simulink model "ex18_sfw_top"  (R2025a)
settings: Solver=FixedStepDiscrete  StartTime=0.0  StopTime=sfw_stop_s  FixedStep=sfw_sample_s  RelTol=1e-3
InitFcn:
  | model_dir = fileparts(get_param(bdroot, 'FileName'));if ~isempty(model_dir), addpath(model_dir); addpath(fullfile(model_dir, 'filterlib')); addpath(fullfile(model_dir, 'dialogs')); end;setup_ex18_sfw;
undefined symbols (not defined in the file or in its folder): gpr_rx_angle_deg, gpr_soil_fir, iq_lo_amp, iq_lo_hz, iq_lpf_num, physconst, rational, rf_z0_ohm, rx_down_if_bpf_den, rx_down_if_bpf_num, S, sfw_freq_hz, sfw_sample_s, sparameters, tap_lo_amp, tap_lo_hz, tap_up_bpf_den, tap_up_bpf_num
libraries: simrfV2elements x4, simrfV2util1 x4, simrfV2_lib x2
settings Model: Creator=31885  LastModifiedBy=31885
settings DataIOCC: SaveFormat=StructureWithTime  ReturnWorkspaceOutputs=off

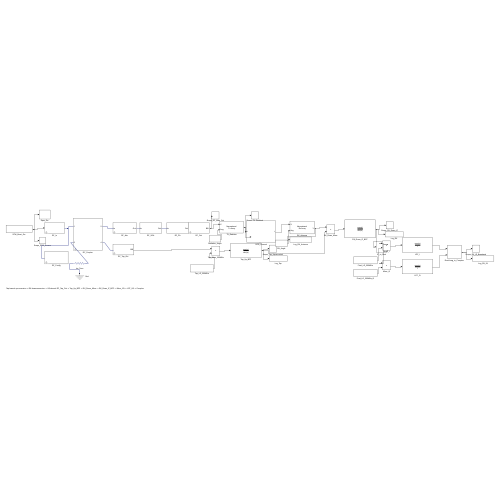
[thumbnail: Simulink's stored preview of the top-level diagram]
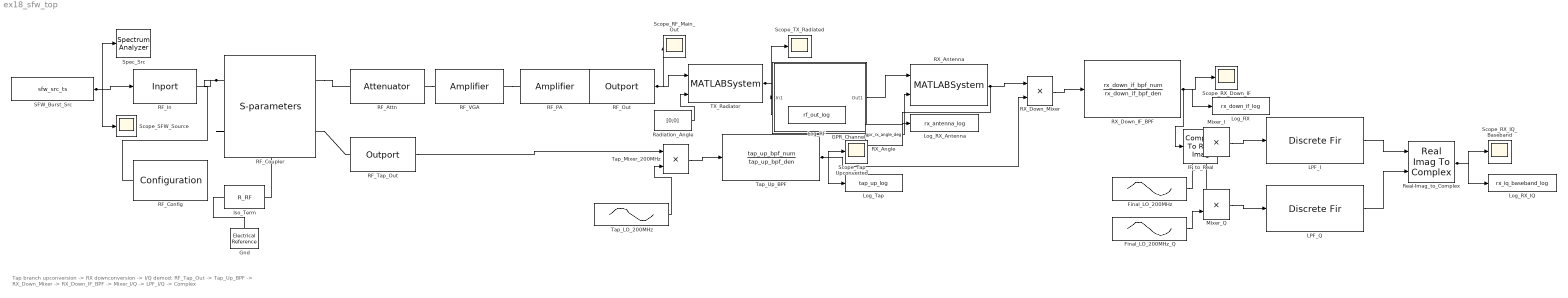
== system ex18_sfw_top ==
  note: Tap branch upconversion -> RX downconversion -> I/Q demod: RF_Tap_Out -> Tap_Up_BPF -> RX_Down_Mixer -> RX_Down_IF_BPF -> Mixer_I/Q -> LPF_I/Q -> Complex
  Final_LO_200MHz : Sin  Amplitude=iq_lo_amp  Frequency=2*pi*iq_lo_hz  SampleTime=sfw_sample_s
  Final_LO_200MHz_Q : Sin  Amplitude=iq_lo_amp  Frequency=2*pi*iq_lo_hz  Phase=-pi/2  SampleTime=sfw_sample_s
  GPR_Channel : Subsystem
  Gnd : simrfV2_lib/Elements/Electrical Reference
      settings: InternalSimscapePortConfiguration="{\"Bottom\":[],\"Left\":[{\"id\":\"V\",\"label\":\"\",\"type\":\"foundation.rf.circuitenvelope\"}],\"Right\":[],\"Top\":[]}"
  IF_to_Real : ComplexToRealImag
  Iso_Term : simrfV2_lib/Elements/R_RF  R=rf_z0_ohm Ohm
      settings: InternalSimscapePortConfiguration="{\"Bottom\":[],\"Left\":[{\"id\":\"p\",\"label\":\"+\",\"type\":\"foundation.rf.circuitenvelope\"}],\"Right\":[{\"id\":\"n\",\"label\":\"-\",\"type\":\"foundation.rf.circuitenvelope\"}],\"Top\":[]}"
  LPF_I : DiscreteFir  Coefficients=iq_lpf_num  SampleTime=sfw_sample_s
      settings: OpenFcn=ex18_filter_dialog(gcb);
  LPF_Q : DiscreteFir  Coefficients=iq_lpf_num  SampleTime=sfw_sample_s
      settings: OpenFcn=ex18_filter_dialog(gcb);
  Log_RF : ToWorkspace  VariableName=rf_out_log  SaveFormat=Structure With Time  SampleTime=-1
  Log_RX : ToWorkspace  VariableName=rx_down_if_log  SaveFormat=Structure With Time  SampleTime=-1
  Log_RX_Antenna : ToWorkspace  VariableName=rx_antenna_log  SaveFormat=Structure With Time  SampleTime=-1
  Log_RX_IQ : ToWorkspace  VariableName=rx_iq_baseband_log  SaveFormat=Structure With Time  SampleTime=-1
  Log_Tap : ToWorkspace  VariableName=tap_up_log  SaveFormat=Structure With Time  SampleTime=-1
  Mixer_I : Product  Inputs=**
  Mixer_Q : Product  Inputs=**
  RF_Attn : simrfV2elements/Attenuator  classname=attenuator  Att=rf_attn_db  Zin=rf_z0_ohm  Zout=rf_z0_ohm  AddNoise=on  InternalGrounding=on
  RF_Config : simrfV2util1/Configuration  AutoFreq=on  Tones=[] Hz  Harmonics=[]  NormalizeCarrierPower=on  SolverType=Auto  UseCCode=on  StepSize=sfw_sample_s s  AddNoise=on  defaultRNG=on  Seed=0  Temperature=290.0 K  SolverDelFlag=0  AbsTol=1e-6  RelTol=1e-3  MaxIter=10  ErrorEstimationType=2-norm over all variables  EnableInterpFilter=on  HiddenFIRfilterControllerParam=off  SmallSignalApprox=off  AllSimFreqs=on  SimFreqs=[] Hz  SimFreqsInternal=[]  SamplesPerFrame=1
  RF_Coupler : simrfV2elements/S-parameters  classname=sparam_element  DataSource=Network-parameters  File=unitygain.s2p  isNetworkObj=off  NetworkObject=sparameters('default.s2p')  Paramtype=S-parameters  Sparam=[0 0 0 0;0.70794578438413791 0 0 0;0 0 0 0;0.50118723362727224 0 0 0]  SparamFreq=145000000 Hz  SparamZ0=50  isRationalObj=off  RationalObject=rational('default.s2p')  Residues=0  Poles=0  DF={0 0; 1 0}  FitOpt=Share all poles  FitTol=-40  MaxPoles=48  SourceFreq=Extracted from data source  PlotFreq=[1e9:1e6:3e9] Hz  PlotType=X-Y plane  YParam1=S(1,1)  YFormat1=Magnitude (dB)  YParam2=None  YFormat2=Magnitude (dB)  YOption=Linear  XOption=Linear  AddNoise=off  InternalGrounding=on  SparamRepresentation=Time domain  AutoImpulseLength=on  ImpulseLength=1e-10 s  MagModeling=off  CacheLevel=0
  RF_In : simrfV2util1/Inport  SimulinkInputSignalType=Ideal voltage  CarrierFreq=0 Hz  ZS=rf_z0_ohm  UseSqWave=off  NumCoeff=10  Bias=0  DutyCyc=50  InternalGrounding=on
  RF_Out : simrfV2util1/Outport  SensorType=Ideal voltage  OutputFormat=Complex Baseband  CarrierFreq=0 Hz  ZL=rf_z0_ohm  InternalGrounding=on  StepSize=sfw_sample_s s  AutoStep=on  HalfPolyphaseLength=12
  RF_PA : simrfV2elements/Amplifier  classname=amplifier  DataSource=Data file  File=unitygain.s2p  isNetworkObj=off  NetworkObject=sparameters('default.s2p')  Paramtype=S-parameters  Sparam=[0 0;1 0]  SparamFreq=1e9 Hz  SparamZ0=50  isRationalObj=off  RationalObject=rational('default.s2p')  Residues=0  Poles=0  DF={0 0; 1 0}  Source_linear_gain=Available power gain  linear_gain=rf_pa_gain_db dB  AmAmAmPmTable=[-25,5,-1;-10,20,-2;0,27,5;5,28,12]  Zin=rf_z0_ohm  Zout=rf_z0_ohm  Source_Poly=Even and odd order  Poly_Coeffs=[0 1]  IPType=Output  IP2=inf dBm  IP3=inf dBm  P1dB=inf dBm  Psat=inf dBm  Gcomp=inf dBm  InternalGrounding=on  SourceFreq=Extracted from data source  PlotFreq=[1e9:1e6:3e9] Hz  PlotType=X-Y plane  YParam1=S(1,1)  YFormat1=Magnitude (dB)  YParam2=None  YFormat2=Magnitude (dB)  YOption=Linear  XOption=Linear  SparamRepresentation=Time domain  FitTol=-40  FitOpt=Fit individually  MaxPoles=48  AutoImpulseLength=on  ImpulseLength=1e-10 s  MagModeling=off  AddNoise=on  NoiseType=Noise figure  NoiseDist=White  NF=rf_pa_nf_db  MinNF=0  Gopt=0  RN=0  CarrierFreq=0 Hz  NoiseAutoImpulseLength=on  NoiseImpulseLength=1e-10 s  ConstS21NL=off  OpFreq=1 GHz  SetOpFreqAsMaxS21=off
  RF_Tap_Out : simrfV2util1/Outport  SensorType=Ideal voltage  OutputFormat=Complex Baseband  CarrierFreq=0 Hz  ZL=rf_z0_ohm  InternalGrounding=on  StepSize=sfw_sample_s s  AutoStep=on  HalfPolyphaseLength=12
  RF_VGA : simrfV2elements/Amplifier  classname=amplifier  DataSource=Data file  File=unitygain.s2p  isNetworkObj=off  NetworkObject=sparameters('default.s2p')  Paramtype=S-parameters  Sparam=[0 0;1 0]  SparamFreq=1e9 Hz  SparamZ0=50  isRationalObj=off  RationalObject=rational('default.s2p')  Residues=0  Poles=0  DF={0 0; 1 0}  Source_linear_gain=Available power gain  linear_gain=rf_vga_gain_db dB  AmAmAmPmTable=[-25,5,-1;-10,20,-2;0,27,5;5,28,12]  Zin=rf_z0_ohm  Zout=rf_z0_ohm  Source_Poly=Even and odd order  Poly_Coeffs=[0 1]  IPType=Output  IP2=inf dBm  IP3=inf dBm  P1dB=inf dBm  Psat=inf dBm  Gcomp=inf dBm  InternalGrounding=on  SourceFreq=Extracted from data source  PlotFreq=[1e9:1e6:3e9] Hz  PlotType=X-Y plane  YParam1=S(1,1)  YFormat1=Magnitude (dB)  YParam2=None  YFormat2=Magnitude (dB)  YOption=Linear  XOption=Linear  SparamRepresentation=Time domain  FitTol=-40  FitOpt=Fit individually  MaxPoles=48  AutoImpulseLength=on  ImpulseLength=1e-10 s  MagModeling=off  AddNoise=on  NoiseType=Noise figure  NoiseDist=White  NF=rf_vga_nf_db  MinNF=0  Gopt=0  RN=0  CarrierFreq=0 Hz  NoiseAutoImpulseLength=on  NoiseImpulseLength=1e-10 s  ConstS21NL=off  OpFreq=1 GHz  SetOpFreqAsMaxS21=off
  RX_Angle : Constant  Value=gpr_rx_angle_deg
  RX_Antenna : MATLABSystem  System=phased.Collector  PropagationSpeed=physconst( 'LightSpeed' )  OperatingFrequency=mean(sfw_freq_hz)  Wavefront=Plane  SensorGainMeasure=dB  Polarization=None  WeightsInputPort=off  SimulateUsing=Code generation  Sensor=phased.IsotropicAntennaElement
      mask Type: phased.Collector
  RX_Down_IF_BPF : DiscreteFilter  Numerator=rx_down_if_bpf_num  Denominator=rx_down_if_bpf_den  SampleTime=sfw_sample_s
      settings: OpenFcn=ex18_filter_dialog(gcb);
  RX_Down_Mixer : Product  Inputs=**
  Radiation_Angle : Constant  Value=[0;0]
  Real-Imag_to_Complex : RealImagToComplex
  SFW_Burst_Src : FromWorkspace  VariableName=sfw_src_ts  SampleTime=sfw_sample_s  Interpolate=off  OutputAfterFinalValue=Holding final value
  Scope_RF_Main_Out : Scope
      settings: DataLoggingVariableName=rf_main_out_log
  Scope_RX_Down_IF : Scope
  Scope_RX_IQ_Baseband : Scope
      settings: DataLoggingVariableName=rx_iq_scope_log
  Scope_SFW_Source : Scope
  Scope_TX_Radiated : Scope
  Scope_Tap_Upconverted : Scope
  Spec_Src : SpectrumAnalyzer  SampleRateSource=Property  SampleRate=sfw_fs_hz  PlotAsTwoSidedSpectrum=off  RBWSource=Property  RBW=100e3  WindowInvariantSamplesPerUpdate=on  FrequencySpan=Start and stop frequencies  StartFrequency=0  StopFrequency=200e6  Title=SFW source spectrum, 0-200 MHz  YLimits=[-100 30]
      settings: OpenAtSimulationStart=off
  TX_Radiator : MATLABSystem  System=phased.Radiator  PropagationSpeed=physconst( 'LightSpeed' )  OperatingFrequency=mean(sfw_freq_hz)  CombineRadiatedSignals=on  SensorGainMeasure=dB  Polarization=None  WeightsInputPort=off  SimulateUsing=Code generation  Sensor=phased.IsotropicAntennaElement
      mask Type: phased.Radiator
  Tap_LO_200MHz : Sin  Amplitude=tap_lo_amp  Frequency=2*pi*tap_lo_hz  SampleTime=sfw_sample_s
  Tap_Mixer_200MHz : Product  Inputs=**
  Tap_Up_BPF : DiscreteFilter  Numerator=tap_up_bpf_num  Denominator=tap_up_bpf_den  SampleTime=sfw_sample_s
      settings: OpenFcn=ex18_filter_dialog(gcb);
  wires:
  SFW_Burst_Src/1 -> RF_In/1, Spec_Src/1, Scope_SFW_Source/1
  RF_Out/1 -> TX_Radiator/1, Scope_RF_Main_Out/1
  Radiation_Angle/1 -> TX_Radiator/2
  TX_Radiator/1 -> Scope_TX_Radiated/1, Log_RF/1, GPR_Channel/1(In1)
  GPR_Channel/1(Out1) -> RX_Antenna/1
  RX_Angle/1 -> RX_Antenna/2
  RX_Antenna/1 -> RX_Down_Mixer/1, Log_RX_Antenna/1
  RF_Tap_Out/1 -> Tap_Mixer_200MHz/1
  Tap_LO_200MHz/1 -> Tap_Mixer_200MHz/2
  Tap_Mixer_200MHz/1 -> Tap_Up_BPF/1
  Tap_Up_BPF/1 -> Scope_Tap_Upconverted/1, Log_Tap/1, RX_Down_Mixer/2
  RX_Down_Mixer/1 -> RX_Down_IF_BPF/1
  RX_Down_IF_BPF/1 -> Scope_RX_Down_IF/1, Log_RX/1, IF_to_Real/1
  IF_to_Real/1 -> Mixer_I/1, Mixer_Q/1
  Final_LO_200MHz/1 -> Mixer_I/2
  Final_LO_200MHz_Q/1 -> Mixer_Q/2
  Mixer_I/1 -> LPF_I/1
  Mixer_Q/1 -> LPF_Q/1
  LPF_I/1 -> Real-Imag_to_Complex/1
  LPF_Q/1 -> Real-Imag_to_Complex/2
  Real-Imag_to_Complex/1 -> Scope_RX_IQ_Baseband/1, Log_RX_IQ/1
  connections:
  RF_Coupler/LConn1 -- RF_In/RConn1 -- RF_Config/LConn1
  RF_Coupler/RConn1 -- RF_Attn/LConn1
  RF_Attn/RConn1 -- RF_VGA/LConn1
  RF_VGA/RConn1 -- RF_PA/LConn1
  RF_PA/RConn1 -- RF_Out/LConn1
  RF_Coupler/RConn2 -- RF_Tap_Out/LConn1
  RF_Coupler/LConn2 -- Iso_Term/RConn1
  Iso_Term/LConn1 -- Gnd/LConn1

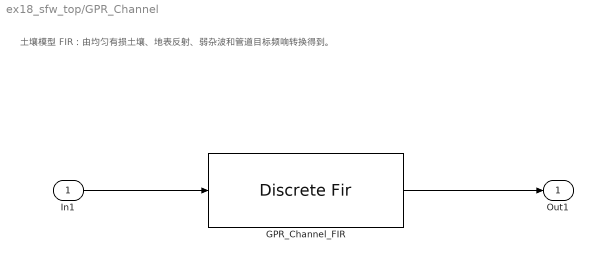
== system ex18_sfw_top/GPR_Channel ==
  note: 土壤模型 FIR：由均匀有损土壤、地表反射、弱杂波和管道目标频响转换得到。
  In1 : Inport
  GPR_Channel_FIR : DiscreteFir  Coefficients=gpr_soil_fir  SampleTime=sfw_sample_s
  Out1 : Outport
  wires:
  In1/1 -> GPR_Channel_FIR/1
  GPR_Channel_FIR/1 -> Out1/1
